simulink model "sim_rectifier"  (R2018a)
settings: Solver=FixedStepAuto  StartTime=0.0  StopTime=11  FixedStep=Ti  RelTol=1e-3
undefined symbols (not defined in the file): A, B, Co, L, opt_constant_reference, opt_dead_time, opt_pwm, opt_pwm_current_controller, opt_theorem, P, pwm_limit_lower, pwm_limit_upper, pwm_period, pwm_pid_kd, pwm_pid_ki, pwm_pid_kp, pwm_pid_vc_ci, pwm_pid_vc_cp, pwm_pid_vc_vi, pwm_pid_vc_vp, pwm_sample_time, Q, R, sensor_sample, sys, Ti, Ts, Vref, x0, xe
libraries: simulink x17, powerlib x13, pePwmGenerator x2, powerlib_meascontrol x1
settings Model: Creator=TARCIO-FEM  LastModifiedBy=Julio-LEPO
settings OptimizationCC: EfficientMapNaN2IntZero=off
settings DebuggingCC: UnconnectedInputMsg=none  UnconnectedOutputMsg=none  UnconnectedLineMsg=none
settings HardwareCC: TargetBitPerPointer=64  TargetBitPerSizeT=64  TargetBitPerPtrDiffT=64  TargetLongLongMode=on  TargetIntDivRoundTo=Zero  TargetEndianess=LittleEndian  TargetWordSize=64  TargetHWDeviceType=MATLAB Host  ProdEqTarget=off
settings CodeAppCC: MaxIdLength=128
settings GRTTargetCC: TargetLangStandard=C89/C90 (ANSI)  CombineOutputUpdateFcns=off  GRTInterface=on

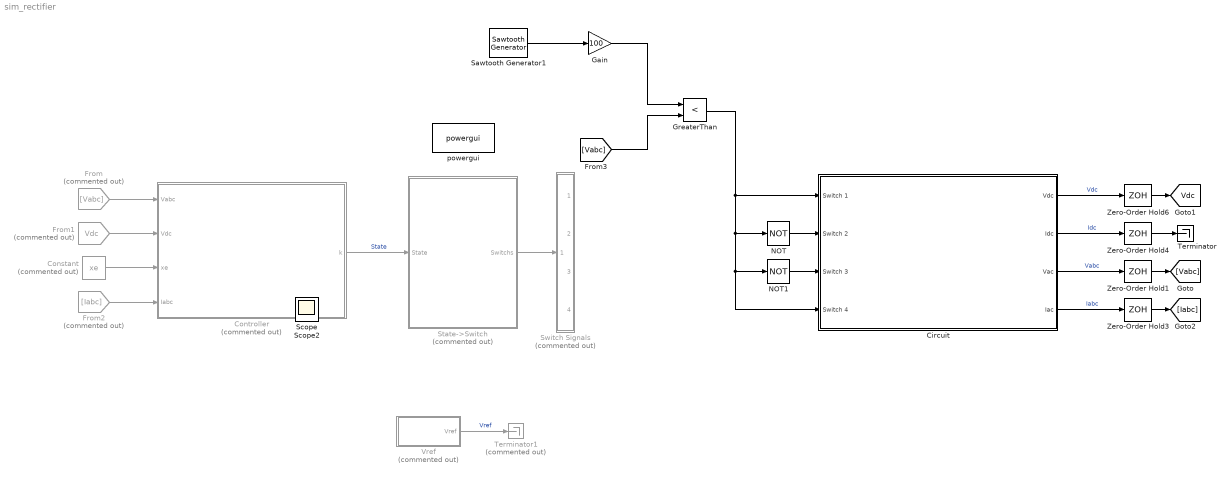
== system sim_rectifier ==
  Circuit : Subsystem
  Constant : Constant  Commented=on  Value=xe
  Controller : Subsystem  Commented=on
  From : From  Commented=on  GotoTag=Vabc
  From1 : From  Commented=on  GotoTag=Vdc  TagVisibility=global
  From2 : From  Commented=on  GotoTag=Iabc
  Gain : Gain  Gain=100
  GreaterThan : RelationalOperator  Operator=<  OutDataTypeStr=boolean  RndMeth=Simplest
  NOT : Logic  Operator=NOT  IconShape=distinctive  AllPortsSameDT=off  OutDataTypeStr=boolean
  NOT1 : Logic  Operator=NOT  IconShape=distinctive  AllPortsSameDT=off  OutDataTypeStr=boolean
  Sawtooth Generator1 : powerlib_meascontrol/Pulse & Signal Generators/Sawtooth Generator  Freq=2e3  Phase=180  Ts=0
      settings: SourceProductName=Simscape Power Systems
  State->Switch : Subsystem  Commented=on
  Switch Signals : Subsystem  Commented=on
  Terminator : Terminator
  Terminator1 : Terminator  Commented=on
  Vref : Subsystem  Commented=on
  Zero-Order Hold{1,3..4,6} (4 alike) : ZeroOrderHold  SampleTime=sensor_sample
  powergui : powerlib/powergui  Priority=1  SimulationMode=Discrete  SampleTime=Ti  frequency=60  Iterations=50  frequencyindice=0  Pbase=100e6  ErrMax=1e-4  UnitsV=kV  UnitsW=MW  buscounter=0  FunctionMessages=off  echomessages=off  EnableUseOfTLC=off  CurrentSourceSwitches=off  DisableSnubberDevices=off  DisableRonSwitches=off  DisableVfSwitches=off  DisplayEquations=off  SolverType=Tustin/Backward Euler (TBE)  Interpol=off  ExternalGateDelay=off  methode=off  Ts=100  x0status=blocks  SPID=off  SwTol=0  HookPort=off  RestoreLinks=warning  ResistiveCurrentMeasurement=off  Frange=[0:2:500]  Ylog=off  Xlog=on  ShowGrid=off  save=off  variable=ZData  structure=0  ZoomFFT=off  StartTime=0.0  cycles=1  DisplayStyle=1  fundamental=60  FreqAxis=off  MaxFrequency=1000  frequencyindicesteady=1  RmsSteady=1  display=off
  Scope : Scope
  Scope2 : Scope
  tag scope: Vdc=global
  wires:
  Controller/1(k) -> State->Switch/1(State)  "State"
  From1/1 -> Controller/2(Vdc)
  Constant/1 -> Controller/3(xe)
  From/1 -> Controller/1(Vabc)
  Vref/1(Vref) -> Terminator1/1  "Vref"
  Zero-Order Hold6/1 -> [Vdc]
  Zero-Order Hold1/1 -> [Vabc]
  Zero-Order Hold3/1 -> [Iabc]
  Circuit/3(Vac) -> Zero-Order Hold1/1  "Vabc"
  Circuit/1(Vdc) -> Zero-Order Hold6/1  "Vdc"
  Circuit/4(Iac) -> Zero-Order Hold3/1  "Iabc"
  State->Switch/1(Switchs) -> Switch Signals/1(In1)
  Zero-Order Hold4/1 -> Terminator/1
  Circuit/2(Idc) -> Zero-Order Hold4/1  "Idc"
  From2/1 -> Controller/4(Iabc)
  GreaterThan/1 -> Circuit/1(Switch 1), Circuit/4(Switch 4), NOT1/1, NOT/1
  NOT/1 -> Circuit/2(Switch 2)
  NOT1/1 -> Circuit/3(Switch 3)
  Sawtooth Generator1/1 -> Gain/1
  [Vabc] -> GreaterThan/2
  Gain/1 -> GreaterThan/1

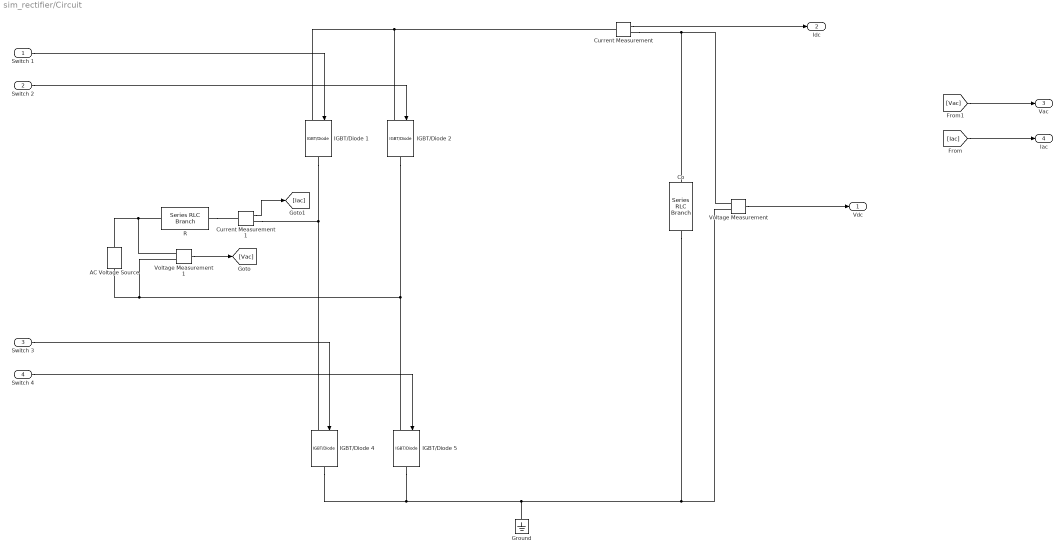
== system sim_rectifier/Circuit ==
  Switch 1 : Inport
  Switch 2 : Inport  Port=2
  Switch 3 : Inport  Port=3
  Switch 4 : Inport  Port=4
  AC Voltage Source : powerlib/Electrical Sources/AC Voltage Source  Amplitude=100  Phase=0  Frequency=60  SampleTime=0  Measurements=None  BusType=swing  Pref=10e3  Qref=0  Qmin=-inf  Qmax=+inf
  Co : powerlib/Elements/Series RLC Branch  LConnTagsString=__new0  RConnTagsString=__new0  BranchType=C  Resistance=R  Inductance=1e-3  SetiL0=off  InitialCurrent=0  Capacitance=Co  Setx0=on  InitialVoltage=x0(1)  Measurements=None
  Current Measurement : powerlib/Measurements/Current Measurement  PhasorSimulation=off  OutputType=Complex  PSBequivalent=0
  Current Measurement1 : powerlib/Measurements/Current Measurement  PhasorSimulation=off  OutputType=Complex  PSBequivalent=0
  Ground : powerlib/Elements/Ground  LConnTagsString=a
  IGBT/Diode {1..2,4..5} (4 alike) : powerlib/Power Electronics/IGBT//Diode  Ron=1e-3  Rs=1e5  Cs=inf  Measurements=off
  R : powerlib/Elements/Series RLC Branch  LConnTagsString=__new0  RConnTagsString=__new0  BranchType=RL  Resistance=R  Inductance=L  SetiL0=off  InitialCurrent=0  Capacitance=1e-6  Setx0=off  InitialVoltage=0  Measurements=None
  Voltage Measurement : powerlib/Measurements/Voltage Measurement  PhasorSimulation=off  OutputType=Complex  PSBequivalent=0
  Voltage Measurement1 : powerlib/Measurements/Voltage Measurement  PhasorSimulation=off  OutputType=Complex  PSBequivalent=0
  Vdc : Outport
  Idc : Outport  Port=2
  Vac : Outport  Port=3
  Iac : Outport  Port=4
  wires:
  Switch 3/1 -> IGBT/Diode 4/1
  Switch 4/1 -> IGBT/Diode 5/1
  Switch 1/1 -> IGBT/Diode 1/1
  Switch 2/1 -> IGBT/Diode 2/1
  Voltage Measurement/1 -> Vdc/1
  [Vac] -> Vac/1
  Current Measurement/1 -> Idc/1
  [Iac] -> Iac/1
  Current Measurement1/1 -> [Iac]
  Voltage Measurement1/1 -> [Vac]
  connections:
  IGBT/Diode 1/RConn1 -- Current Measurement1/RConn1 -- IGBT/Diode 4/LConn1
  Voltage Measurement/LConn1 -- Current Measurement/RConn1 -- Co/LConn1
  Co/RConn1 -- Voltage Measurement/LConn2 -- IGBT/Diode 4/RConn1 -- IGBT/Diode 5/RConn1 -- Ground/LConn1
  Current Measurement/LConn1 -- IGBT/Diode 1/LConn1 -- IGBT/Diode 2/LConn1
  IGBT/Diode 2/RConn1 -- Voltage Measurement1/LConn2 -- AC Voltage Source/LConn1 -- IGBT/Diode 5/LConn1
  AC Voltage Source/RConn1 -- R/LConn1 -- Voltage Measurement1/LConn1
  R/RConn1 -- Current Measurement1/LConn1

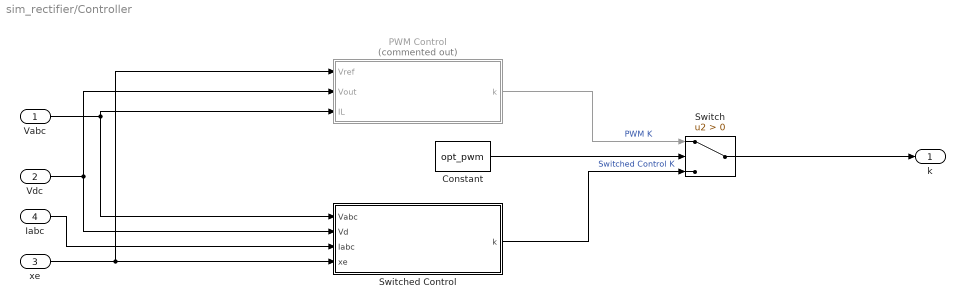
== system sim_rectifier/Controller ==
  Vabc : Inport
  Vdc : Inport  Port=2
  xe : Inport  Port=3
  Iabc : Inport  Port=4
  Constant : Constant  Value=opt_pwm
  PWM Control : Subsystem  Commented=on
  Switch : Switch  Criteria=u2 > Threshold
  Switched Control : Subsystem
  k : Outport
  wires:
  Vabc/1 -> PWM Control/3(IL), Switched Control/1(Vabc)
  Vdc/1 -> PWM Control/2(Vout), Switched Control/2(Vd)
  PWM Control/1(k) -> Switch/1  "PWM K"
  Switched Control/1(k) -> Switch/3  "Switched Control K"
  Constant/1 -> Switch/2
  xe/1 -> PWM Control/1(Vref), Switched Control/4(xe)
  Switch/1 -> k/1
  Iabc/1 -> Switched Control/3(Iabc)

== system sim_rectifier/State->Switch ==
  State : Inport
  Rectifier : Subsystem
  Switchs : Outport
  wires:
  Rectifier/1(Switchs) -> Switchs/1  "Switch Signal"
  State/1 -> Rectifier/1(State)

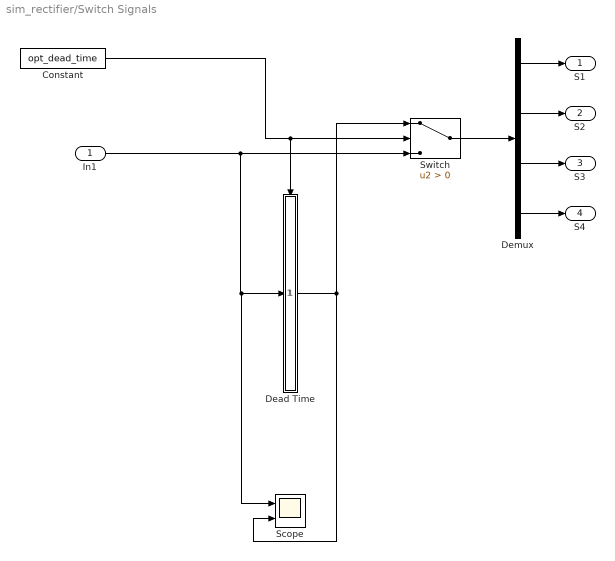
== system sim_rectifier/Switch Signals ==
  In1 : Inport
  Constant : Constant  Value=opt_dead_time
  Dead Time : Subsystem
  Demux : Demux
  Scope : Scope  NumInputPorts=2
  Switch : Switch  Criteria=u2 > Threshold
  S1 : Outport
  S2 : Outport  Port=2
  S3 : Outport  Port=3
  S4 : Outport  Port=4
  wires:
  Constant/1 -> Dead Time/Enable, Switch/2
  Dead Time/1(Out1) -> Scope/2, Switch/1
  In1/1 -> Scope/1, Dead Time/1(In1), Switch/3
  Demux/2 -> S2/1
  Demux/1 -> S1/1
  Demux/4 -> S4/1
  Demux/3 -> S3/1
  Switch/1 -> Demux/1

== system sim_rectifier/Vref ==
  Constant Reference : Subsystem
  Switch1 : Switch  Criteria=u2 > Threshold
  Variable Reference : Subsystem
  opt_constant_reference : Constant  Value=opt_constant_reference
  Vref : Outport
  wires:
  opt_constant_reference/1 -> Switch1/2
  Switch1/1 -> Vref/1
  Variable Reference/1(Vref) -> Switch1/3
  Constant Reference/1(Vref) -> Switch1/1

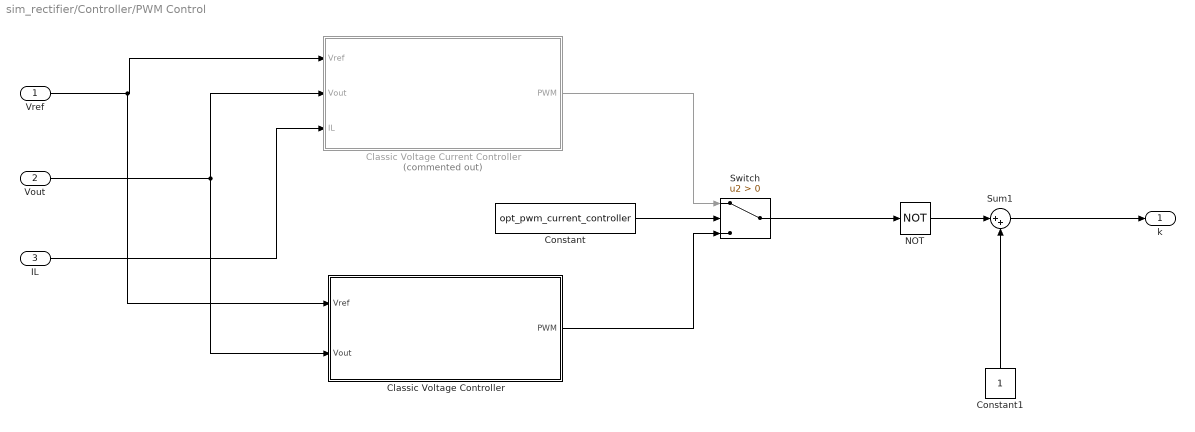
== system sim_rectifier/Controller/PWM Control ==
  Vref : Inport
  Vout : Inport  Port=2
  IL : Inport  Port=3
  Classic Voltage Controller : Subsystem
  Classic Voltage Current Controller : Subsystem  Commented=on
  Constant : Constant  Value=opt_pwm_current_controller
  Constant1 : Constant
  NOT : Logic  Operator=NOT  IconShape=distinctive  AllPortsSameDT=off  OutDataTypeStr=boolean
  Sum1 : Sum  Inputs=|++
  Switch : Switch  Criteria=u2 > Threshold
  k : Outport
  wires:
  Sum1/1 -> k/1
  NOT/1 -> Sum1/1
  Constant1/1 -> Sum1/2
  Vref/1 -> Classic Voltage Controller/1(Vref), Classic Voltage Current Controller/1(Vref)
  Vout/1 -> Classic Voltage Controller/2(Vout), Classic Voltage Current Controller/2(Vout)
  IL/1 -> Classic Voltage Current Controller/3(IL)
  Constant/1 -> Switch/2
  Classic Voltage Controller/1(PWM) -> Switch/3
  Classic Voltage Current Controller/1(PWM) -> Switch/1
  Switch/1 -> NOT/1

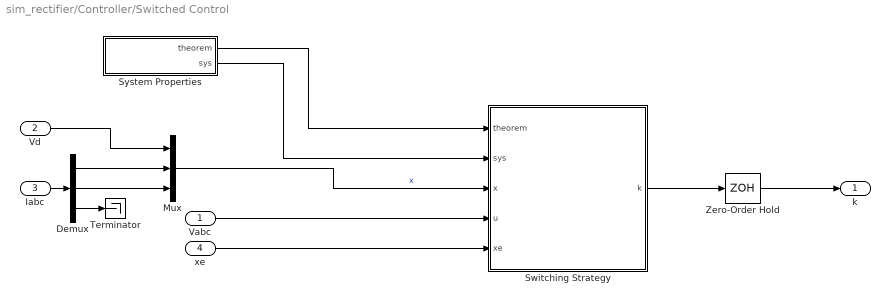
== system sim_rectifier/Controller/Switched Control ==
  Vabc : Inport
  Vd : Inport  Port=2
  Iabc : Inport  Port=3
  xe : Inport  Port=4
  Demux : Demux  Outputs=3
  Mux : Mux  Inputs=3
  Switching Strategy : MATLAB Function  TreatAsAtomicUnit=on
  System Properties : Subsystem
  Terminator : Terminator
  Zero-Order Hold : ZeroOrderHold  SampleTime=Ts
  k : Outport
  wires:
  Switching Strategy/1(k) -> Zero-Order Hold/1
  System Properties/2(sys) -> Switching Strategy/2(sys)
  Vabc/1 -> Switching Strategy/4(u)
  xe/1 -> Switching Strategy/5(xe)
  Zero-Order Hold/1 -> k/1
  System Properties/1(theorem) -> Switching Strategy/1(theorem)
  Iabc/1 -> Demux/1
  Demux/3 -> Terminator/1
  Demux/2 -> Mux/3
  Demux/1 -> Mux/2
  Vd/1 -> Mux/1
  Mux/1 -> Switching Strategy/3(x)  "x"

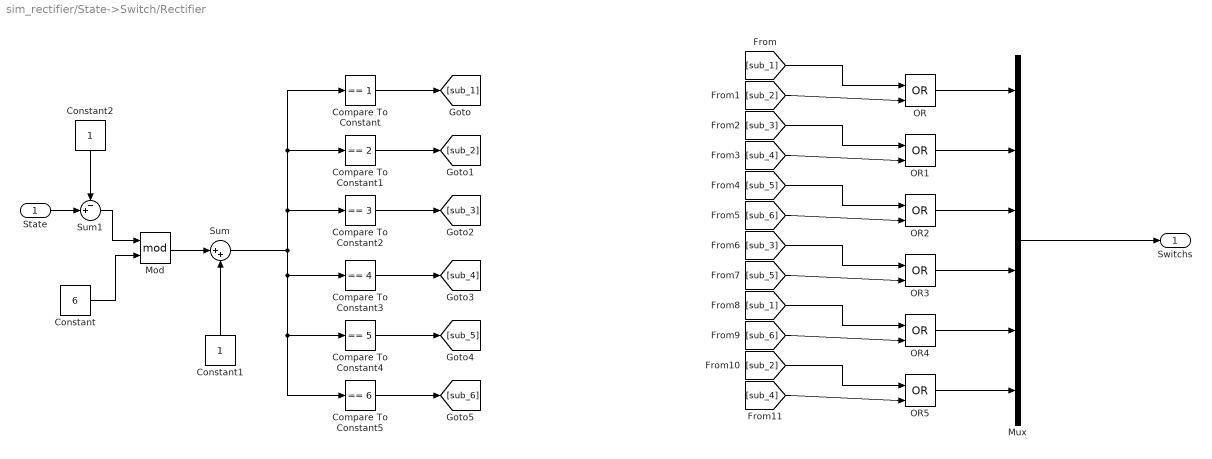
== system sim_rectifier/State->Switch/Rectifier ==
  State : Inport
  Compare To Constant : simulink/Logic and Bit Operations/Compare To Constant  relop===  const=1  OutDataTypeStr=boolean
  Compare To Constant1 : simulink/Logic and Bit Operations/Compare To Constant  relop===  const=2  OutDataTypeStr=boolean
  Compare To Constant2 : simulink/Logic and Bit Operations/Compare To Constant  relop===  const=3  OutDataTypeStr=boolean
  Compare To Constant3 : simulink/Logic and Bit Operations/Compare To Constant  relop===  const=4  OutDataTypeStr=boolean
  Compare To Constant4 : simulink/Logic and Bit Operations/Compare To Constant  relop===  const=5  OutDataTypeStr=boolean
  Compare To Constant5 : simulink/Logic and Bit Operations/Compare To Constant  relop===  const=6  OutDataTypeStr=boolean
  Constant : Constant  Value=6
  Constant1 : Constant
  Constant2 : Constant
  Mod : Math  Operator=mod  SaturateOnIntegerOverflow=on
  Mux : Mux  Inputs=6
  OR{,1..5} (6 alike) : Logic  Operator=OR  IconShape=distinctive  AllPortsSameDT=off  OutDataTypeStr=boolean
  Sum : Sum  Inputs=|++
  Sum1 : Sum  Inputs=-+|
  Switchs : Outport
  wires:
  Mux/1 -> Switchs/1
  [sub_1] -> OR/1
  [sub_2] -> OR/2
  Compare To Constant/1 -> [sub_1]
  Compare To Constant2/1 -> [sub_3]
  OR/1 -> Mux/1
  Compare To Constant1/1 -> [sub_2]
  Compare To Constant3/1 -> [sub_4]
  Compare To Constant4/1 -> [sub_5]
  Compare To Constant5/1 -> [sub_6]
  [sub_4] -> OR1/2
  [sub_3] -> OR1/1
  OR1/1 -> Mux/2
  [sub_6] -> OR2/2
  [sub_5] -> OR2/1
  [sub_5] -> OR3/2
  [sub_3] -> OR3/1
  OR3/1 -> Mux/4
  [sub_6] -> OR4/2
  [sub_1] -> OR4/1
  [sub_4] -> OR5/2
  [sub_2] -> OR5/1
  OR5/1 -> Mux/6
  OR4/1 -> Mux/5
  OR2/1 -> Mux/3
  Constant/1 -> Mod/2
  Mod/1 -> Sum/1
  Sum/1 -> Compare To Constant5/1, Compare To Constant4/1, Compare To Constant3/1, Compare To Constant/1, Compare To Constant1/1, Compare To Constant2/1
  Constant1/1 -> Sum/2
  State/1 -> Sum1/2
  Sum1/1 -> Mod/1
  Constant2/1 -> Sum1/1

== system sim_rectifier/Switch Signals/Dead Time ==
  In1 : Inport
  Enable : EnablePort
  Dead Time : Subsystem
  Dead Time1 : Subsystem
  Dead Time2 : Subsystem
  Dead Time3 : Subsystem
  Demux : Demux
  Mux : Mux
  Out1 : Outport
  wires:
  Demux/4 -> Dead Time3/1(Signal)
  Demux/3 -> Dead Time2/1(Signal)
  Demux/2 -> Dead Time1/1(Signal)
  Demux/1 -> Dead Time/1(Signal)
  In1/1 -> Demux/1
  Dead Time3/1(Signal Delayed) -> Mux/4
  Dead Time2/1(Signal Delayed) -> Mux/3
  Dead Time1/1(Signal Delayed) -> Mux/2
  Dead Time/1(Signal Delayed) -> Mux/1
  Mux/1 -> Out1/1

== system sim_rectifier/Vref/Constant Reference ==
  Constant : Constant  Value=Vref
  Vref : Outport
  wires:
  Constant/1 -> Vref/1

== system sim_rectifier/Vref/Variable Reference ==
  Constant : Constant  Value=Vref
  Rate Limiter : RateLimiter  RisingSlewLimit=10  FallingSlewLimit=-10  SampleTimeMode=inherited
  Step : Step  Time=1.5  After=20  SampleTime=0
  Sum : Sum  Inputs=|++
  Vref : Outport
  wires:
  Constant/1 -> Sum/1
  Sum/1 -> Vref/1
  Step/1 -> Rate Limiter/1
  Rate Limiter/1 -> Sum/2

== system sim_rectifier/Controller/PWM Control/Classic Voltage Controller ==
  Vref : Inport
  Vout : Inport  Port=2
  PID Controller : simulink/Continuous/PID Controller  Controller=PI  TimeDomain=Discrete-time  SampleTime=pwm_period  IntegratorMethod=Forward Euler  FilterMethod=Forward Euler  Form=Parallel  UseFilter=on  ControllerParametersSource=internal  P=pwm_pid_kp  I=pwm_pid_ki  D=pwm_pid_kd  N=100  InitialConditionSource=internal  InitialConditionForIntegrator=0  InitialConditionForFilter=0  ExternalReset=none  LimitOutput=off  UpperSaturationLimit=inf  LowerSaturationLimit=-inf  LinearizeAsGain=on  AntiWindupMode=none  Kb=1  TrackingMode=off  Kt=1  PParamMin=[]  PParamMax=[]  IParamMin=[]  IParamMax=[]  DParamMin=[]  DParamMax=[]  NParamMin=[]  NParamMax=[]  KbParamMin=[]  KbParamMax=[]  KtParamMin=[]  KtParamMax=[]  POutMin=[]  POutMax=[]  IOutMin=[]  IOutMax=[]  DOutMin=[]  DOutMax=[]  NOutMin=[]  NOutMax=[]  KbOutMin=[]  KbOutMax=[]  KtOutMin=[]  KtOutMax=[]  IntegratorOutMin=[]  IntegratorOutMax=[]  FilterOutMin=[]  FilterOutMax=[]  SumOutMin=[]  SumOutMax=[]  SumI1OutMin=[]  SumI1OutMax=[]  SumI2OutMin=[]  SumI2OutMax=[]  SumI3OutMin=[]  SumI3OutMax=[]  SumDOutMin=[]  SumDOutMax=[]  SaturationOutMin=[]  SaturationOutMax=[]  IntegratorContinuousStateAttributes=''  IntegratorStateMustResolveToSignalObject=off  IntegratorRTWStateStorageClass=Auto  FilterContinuousStateAttributes=''  FilterStateMustResolveToSignalObject=off  FilterRTWStateStorageClass=Auto  DifferentiatorICPrevScaledInput=0  DifferentiatorOutMin=[]  DifferentiatorOutMax=[]  FilterDiffOutCoefMin=[]  FilterDiffOutCoefMax=[]  SumDenOutMin=[]  SumDenOutMax=[]  SumNumOutMin=[]  SumNumOutMax=[]  ReciprocalOutMin=[]  ReciprocalOutMax=[]  DivideOutMin=[]  DivideOutMax=[]  TunerSelectOption=Transfer Function Based (PID Tuner App)
  PWM Generator : pePwmGenerator/PWM Generator  CarrCount=Up  Tper=pwm_period  Ts=pwm_sample_time
  Saturation : Saturate  UpperLimit=pwm_limit_upper  LowerLimit=pwm_limit_lower
  Sum : Sum  Inputs=|+-
  PWM : Outport
  wires:
  Saturation/1 -> PWM Generator/1  "PWM Duty Cycle"
  PWM Generator/1 -> PWM/1
  Sum/1 -> PID Controller/1
  Vref/1 -> Sum/1
  Vout/1 -> Sum/2
  PID Controller/1 -> Saturation/1

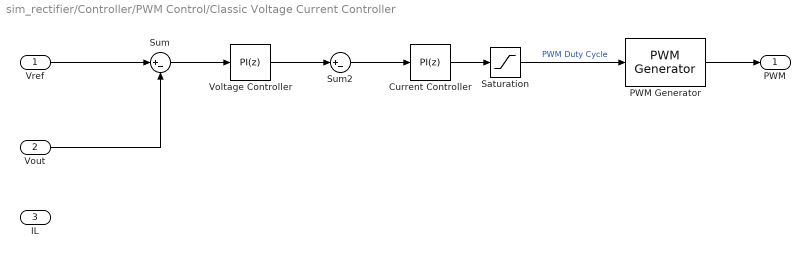
== system sim_rectifier/Controller/PWM Control/Classic Voltage Current Controller ==
  Vref : Inport
  Vout : Inport  Port=2
  IL : Inport  Port=3
  Current Controller : simulink/Continuous/PID Controller  Controller=PI  TimeDomain=Discrete-time  SampleTime=pwm_period  IntegratorMethod=Forward Euler  FilterMethod=Forward Euler  Form=Parallel  UseFilter=on  ControllerParametersSource=internal  P=pwm_pid_vc_cp  I=pwm_pid_vc_ci  D=pwm_pid_kd  N=100  InitialConditionSource=internal  InitialConditionForIntegrator=0  InitialConditionForFilter=0  ExternalReset=none  LimitOutput=off  UpperSaturationLimit=inf  LowerSaturationLimit=-inf  LinearizeAsGain=on  AntiWindupMode=none  Kb=1  TrackingMode=off  Kt=1  PParamMin=[]  PParamMax=[]  IParamMin=[]  IParamMax=[]  DParamMin=[]  DParamMax=[]  NParamMin=[]  NParamMax=[]  KbParamMin=[]  KbParamMax=[]  KtParamMin=[]  KtParamMax=[]  POutMin=[]  POutMax=[]  IOutMin=[]  IOutMax=[]  DOutMin=[]  DOutMax=[]  NOutMin=[]  NOutMax=[]  KbOutMin=[]  KbOutMax=[]  KtOutMin=[]  KtOutMax=[]  IntegratorOutMin=[]  IntegratorOutMax=[]  FilterOutMin=[]  FilterOutMax=[]  SumOutMin=[]  SumOutMax=[]  SumI1OutMin=[]  SumI1OutMax=[]  SumI2OutMin=[]  SumI2OutMax=[]  SumI3OutMin=[]  SumI3OutMax=[]  SumDOutMin=[]  SumDOutMax=[]  SaturationOutMin=[]  SaturationOutMax=[]  IntegratorContinuousStateAttributes=''  IntegratorStateMustResolveToSignalObject=off  IntegratorRTWStateStorageClass=Auto  FilterContinuousStateAttributes=''  FilterStateMustResolveToSignalObject=off  FilterRTWStateStorageClass=Auto  DifferentiatorICPrevScaledInput=0  DifferentiatorOutMin=[]  DifferentiatorOutMax=[]  FilterDiffOutCoefMin=[]  FilterDiffOutCoefMax=[]  SumDenOutMin=[]  SumDenOutMax=[]  SumNumOutMin=[]  SumNumOutMax=[]  ReciprocalOutMin=[]  ReciprocalOutMax=[]  DivideOutMin=[]  DivideOutMax=[]  TunerSelectOption=Transfer Function Based (PID Tuner App)
  PWM Generator : pePwmGenerator/PWM Generator  CarrCount=Up  Tper=pwm_period  Ts=pwm_sample_time
  Saturation : Saturate  UpperLimit=pwm_limit_upper  LowerLimit=pwm_limit_lower
  Sum : Sum  Inputs=|+-
  Sum2 : Sum  Inputs=|+-
  Voltage Controller : simulink/Continuous/PID Controller  Controller=PI  TimeDomain=Discrete-time  SampleTime=pwm_period  IntegratorMethod=Forward Euler  FilterMethod=Forward Euler  Form=Parallel  UseFilter=on  ControllerParametersSource=internal  P=pwm_pid_vc_vp  I=pwm_pid_vc_vi  D=0  N=100  InitialConditionSource=internal  InitialConditionForIntegrator=0  InitialConditionForFilter=0  ExternalReset=none  LimitOutput=off  UpperSaturationLimit=inf  LowerSaturationLimit=-inf  LinearizeAsGain=on  AntiWindupMode=none  Kb=1  TrackingMode=off  Kt=1  PParamMin=[]  PParamMax=[]  IParamMin=[]  IParamMax=[]  DParamMin=[]  DParamMax=[]  NParamMin=[]  NParamMax=[]  KbParamMin=[]  KbParamMax=[]  KtParamMin=[]  KtParamMax=[]  POutMin=[]  POutMax=[]  IOutMin=[]  IOutMax=[]  DOutMin=[]  DOutMax=[]  NOutMin=[]  NOutMax=[]  KbOutMin=[]  KbOutMax=[]  KtOutMin=[]  KtOutMax=[]  IntegratorOutMin=[]  IntegratorOutMax=[]  FilterOutMin=[]  FilterOutMax=[]  SumOutMin=[]  SumOutMax=[]  SumI1OutMin=[]  SumI1OutMax=[]  SumI2OutMin=[]  SumI2OutMax=[]  SumI3OutMin=[]  SumI3OutMax=[]  SumDOutMin=[]  SumDOutMax=[]  SaturationOutMin=[]  SaturationOutMax=[]  IntegratorContinuousStateAttributes=''  IntegratorStateMustResolveToSignalObject=off  IntegratorRTWStateStorageClass=Auto  FilterContinuousStateAttributes=''  FilterStateMustResolveToSignalObject=off  FilterRTWStateStorageClass=Auto  DifferentiatorICPrevScaledInput=0  DifferentiatorOutMin=[]  DifferentiatorOutMax=[]  FilterDiffOutCoefMin=[]  FilterDiffOutCoefMax=[]  SumDenOutMin=[]  SumDenOutMax=[]  SumNumOutMin=[]  SumNumOutMax=[]  ReciprocalOutMin=[]  ReciprocalOutMax=[]  DivideOutMin=[]  DivideOutMax=[]  TunerSelectOption=Transfer Function Based (PID Tuner App)
  PWM : Outport
  wires:
  Sum2/1 -> Current Controller/1
  Sum/1 -> Voltage Controller/1
  Vout/1 -> Sum/2
  Voltage Controller/1 -> Sum2/1
  Current Controller/1 -> Saturation/1
  Vref/1 -> Sum/1
  Saturation/1 -> PWM Generator/1  "PWM Duty Cycle"
  PWM Generator/1 -> PWM/1

== system sim_rectifier/Controller/Switched Control/System Properties ==
  Bus Creator : BusCreator  Inputs=5  OutDataTypeStr=Bus: SystemDataBus
  Constant : Constant  Value=A  VectorParams1D=off
  Constant1 : Constant  Value=B  VectorParams1D=off
  Constant2 : Constant  Value=P  VectorParams1D=off
  Constant3 : Constant  Value=Q  VectorParams1D=off
  Constant5 : Constant  Value=sys.N
  Constant6 : Constant  Value=opt_theorem
  theorem : Outport
  sys : Outport  Port=2
  wires:
  Bus Creator/1 -> sys/1
  Constant2/1 -> Bus Creator/3  "P"
  Constant1/1 -> Bus Creator/2  "B"
  Constant/1 -> Bus Creator/1  "A"
  Constant3/1 -> Bus Creator/4  "Q"
  Constant5/1 -> Bus Creator/5  "N"
  Constant6/1 -> theorem/1

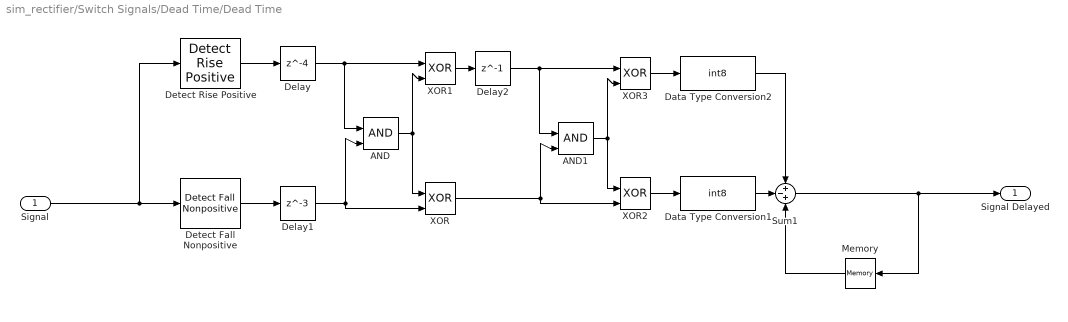
== system sim_rectifier/Switch Signals/Dead Time/Dead Time ==
  Signal : Inport
  AND : Logic  IconShape=distinctive  AllPortsSameDT=off  OutDataTypeStr=boolean
  AND1 : Logic  IconShape=distinctive  AllPortsSameDT=off  OutDataTypeStr=boolean
  Data Type Conversion1 : DataTypeConversion  OutDataTypeStr=int8
  Data Type Conversion2 : DataTypeConversion  OutDataTypeStr=int8
  Delay : Delay  DelayLength=4
  Delay1 : Delay  DelayLength=3
  Delay2 : Delay  DelayLength=1
  Detect Fall Nonpositive : simulink/Logic and Bit Operations/Detect Fall Nonpositive  vinit=true  OutDataTypeStr=boolean
      settings: SourceProductName=Simulink  SourceProductBaseCode=SL
  Detect Rise Positive : simulink/Logic and Bit Operations/Detect Rise Positive  vinit=0  OutDataTypeStr=boolean
  Memory : Memory  InheritSampleTime=on  LinearizeAsDelay=on
  Sum1 : Sum  Inputs=+-+
  XOR{,1..3} (4 alike) : Logic  Operator=XOR  IconShape=distinctive  AllPortsSameDT=off  OutDataTypeStr=boolean
  Signal Delayed : Outport
  wires:
  Sum1/1 -> Memory/1, Signal Delayed/1
  Data Type Conversion1/1 -> Sum1/2
  Memory/1 -> Sum1/3
  Signal/1 -> Detect Fall Nonpositive/1, Detect Rise Positive/1
  Data Type Conversion2/1 -> Sum1/1
  Detect Fall Nonpositive/1 -> Delay1/1
  Detect Rise Positive/1 -> Delay/1
  Delay1/1 -> XOR/2, AND/2
  Delay/1 -> XOR1/1, AND/1
  XOR1/1 -> Delay2/1
  AND/1 -> XOR1/2, XOR/1
  Delay2/1 -> XOR3/1, AND1/1
  AND1/1 -> XOR3/2, XOR2/1
  XOR/1 -> XOR2/2, AND1/2
  XOR3/1 -> Data Type Conversion2/1
  XOR2/1 -> Data Type Conversion1/1

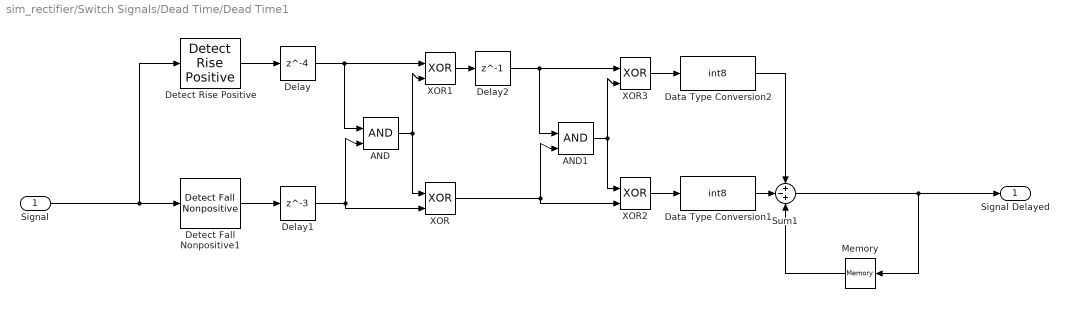
== system sim_rectifier/Switch Signals/Dead Time/Dead Time1 ==
  Signal : Inport
  AND : Logic  IconShape=distinctive  AllPortsSameDT=off  OutDataTypeStr=boolean
  AND1 : Logic  IconShape=distinctive  AllPortsSameDT=off  OutDataTypeStr=boolean
  Data Type Conversion1 : DataTypeConversion  OutDataTypeStr=int8
  Data Type Conversion2 : DataTypeConversion  OutDataTypeStr=int8
  Delay : Delay  DelayLength=4
  Delay1 : Delay  DelayLength=3
  Delay2 : Delay  DelayLength=1
  Detect Fall Nonpositive1 : simulink/Logic and Bit Operations/Detect Fall Nonpositive  vinit=true  OutDataTypeStr=boolean
      settings: SourceProductName=Simulink  SourceProductBaseCode=SL
  Detect Rise Positive : simulink/Logic and Bit Operations/Detect Rise Positive  vinit=0  OutDataTypeStr=boolean
  Memory : Memory  InheritSampleTime=on  LinearizeAsDelay=on
  Sum1 : Sum  Inputs=+-+
  XOR{,1..3} (4 alike) : Logic  Operator=XOR  IconShape=distinctive  AllPortsSameDT=off  OutDataTypeStr=boolean
  Signal Delayed : Outport
  wires:
  Sum1/1 -> Memory/1, Signal Delayed/1
  Data Type Conversion1/1 -> Sum1/2
  Memory/1 -> Sum1/3
  Signal/1 -> Detect Fall Nonpositive1/1, Detect Rise Positive/1
  Data Type Conversion2/1 -> Sum1/1
  Detect Fall Nonpositive1/1 -> Delay1/1
  Detect Rise Positive/1 -> Delay/1
  Delay1/1 -> XOR/2, AND/2
  Delay/1 -> XOR1/1, AND/1
  XOR1/1 -> Delay2/1
  AND/1 -> XOR1/2, XOR/1
  Delay2/1 -> XOR3/1, AND1/1
  AND1/1 -> XOR3/2, XOR2/1
  XOR/1 -> XOR2/2, AND1/2
  XOR3/1 -> Data Type Conversion2/1
  XOR2/1 -> Data Type Conversion1/1

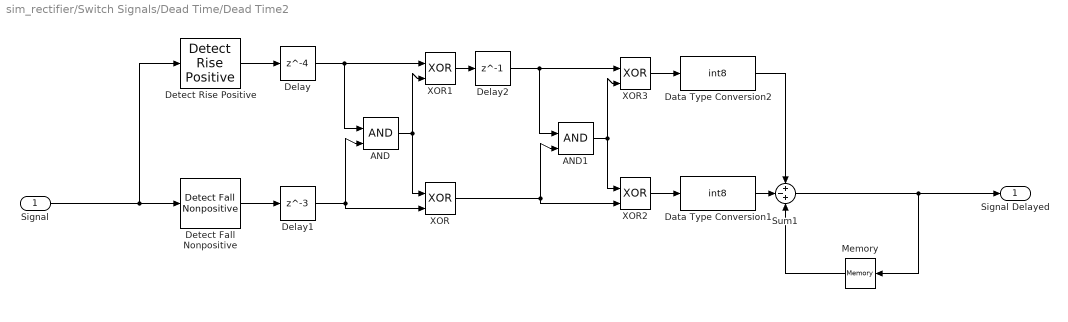
== system sim_rectifier/Switch Signals/Dead Time/Dead Time2 ==
  Signal : Inport
  AND : Logic  IconShape=distinctive  AllPortsSameDT=off  OutDataTypeStr=boolean
  AND1 : Logic  IconShape=distinctive  AllPortsSameDT=off  OutDataTypeStr=boolean
  Data Type Conversion1 : DataTypeConversion  OutDataTypeStr=int8
  Data Type Conversion2 : DataTypeConversion  OutDataTypeStr=int8
  Delay : Delay  DelayLength=4
  Delay1 : Delay  DelayLength=3
  Delay2 : Delay  DelayLength=1
  Detect Fall Nonpositive : simulink/Logic and Bit Operations/Detect Fall Nonpositive  vinit=true  OutDataTypeStr=boolean
      settings: SourceProductName=Simulink  SourceProductBaseCode=SL
  Detect Rise Positive : simulink/Logic and Bit Operations/Detect Rise Positive  vinit=0  OutDataTypeStr=boolean
  Memory : Memory  InheritSampleTime=on  LinearizeAsDelay=on
  Sum1 : Sum  Inputs=+-+
  XOR{,1..3} (4 alike) : Logic  Operator=XOR  IconShape=distinctive  AllPortsSameDT=off  OutDataTypeStr=boolean
  Signal Delayed : Outport
  wires:
  Sum1/1 -> Memory/1, Signal Delayed/1
  Data Type Conversion1/1 -> Sum1/2
  Memory/1 -> Sum1/3
  Signal/1 -> Detect Fall Nonpositive/1, Detect Rise Positive/1
  Data Type Conversion2/1 -> Sum1/1
  Detect Fall Nonpositive/1 -> Delay1/1
  Detect Rise Positive/1 -> Delay/1
  Delay1/1 -> XOR/2, AND/2
  Delay/1 -> XOR1/1, AND/1
  XOR1/1 -> Delay2/1
  AND/1 -> XOR1/2, XOR/1
  Delay2/1 -> XOR3/1, AND1/1
  AND1/1 -> XOR3/2, XOR2/1
  XOR/1 -> XOR2/2, AND1/2
  XOR3/1 -> Data Type Conversion2/1
  XOR2/1 -> Data Type Conversion1/1

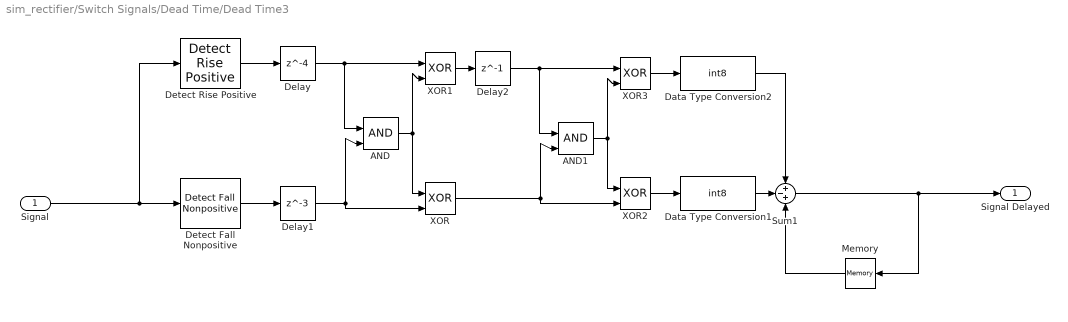
== system sim_rectifier/Switch Signals/Dead Time/Dead Time3 ==
  Signal : Inport
  AND : Logic  IconShape=distinctive  AllPortsSameDT=off  OutDataTypeStr=boolean
  AND1 : Logic  IconShape=distinctive  AllPortsSameDT=off  OutDataTypeStr=boolean
  Data Type Conversion1 : DataTypeConversion  OutDataTypeStr=int8
  Data Type Conversion2 : DataTypeConversion  OutDataTypeStr=int8
  Delay : Delay  DelayLength=4
  Delay1 : Delay  DelayLength=3
  Delay2 : Delay  DelayLength=1
  Detect Fall Nonpositive : simulink/Logic and Bit Operations/Detect Fall Nonpositive  vinit=true  OutDataTypeStr=boolean
      settings: SourceProductName=Simulink  SourceProductBaseCode=SL
  Detect Rise Positive : simulink/Logic and Bit Operations/Detect Rise Positive  vinit=0  OutDataTypeStr=boolean
  Memory : Memory  InheritSampleTime=on  LinearizeAsDelay=on
  Sum1 : Sum  Inputs=+-+
  XOR{,1..3} (4 alike) : Logic  Operator=XOR  IconShape=distinctive  AllPortsSameDT=off  OutDataTypeStr=boolean
  Signal Delayed : Outport
  wires:
  Sum1/1 -> Memory/1, Signal Delayed/1
  Data Type Conversion1/1 -> Sum1/2
  Memory/1 -> Sum1/3
  Signal/1 -> Detect Rise Positive/1, Detect Fall Nonpositive/1
  Data Type Conversion2/1 -> Sum1/1
  Detect Fall Nonpositive/1 -> Delay1/1
  Detect Rise Positive/1 -> Delay/1
  Delay1/1 -> XOR/2, AND/2
  Delay/1 -> XOR1/1, AND/1
  XOR1/1 -> Delay2/1
  AND/1 -> XOR1/2, XOR/1
  Delay2/1 -> XOR3/1, AND1/1
  AND1/1 -> XOR3/2, XOR2/1
  XOR/1 -> XOR2/2, AND1/2
  XOR3/1 -> Data Type Conversion2/1
  XOR2/1 -> Data Type Conversion1/1

== matlab function sim_rectifier/Controller/Switched Control/Switching Strategy ==
  data: theorem input; sys input; x input; u input; k output; xe input
function k = switching_strategy(theorem, sys, x, u, xe)
    N = 3;
    qsi = x - xe;
    sig = inf(N,1);
    
    for i=1:N
        j = i;
        if any(i==[4 6])
            if x(2) < 0
                j = i+6;
            end
        elseif any(i==[2 5])
            if x(3) < 0
                j = i+6;
            end
        else
            if -x(2)-x(3) < 0
                j = i+6;
            end
        end
        
        switch(theorem)
            case 1
                sig(i) = qsi'*(sys.Q(:,:,j)*qsi + 2*sys.P*(sys.A(:,:,j)*x + sys.B(:,:,j)*u));
            case 2
                sig(i) = qsi'*sys.P*(sys.A(:,:,j)*xe + sys.B(:,:,j)*u);
        end
    end
    [~, k] = min(sig);
end
